simulink model "TwoD_Missile_Target"  (R2020b)
settings: Solver=ode4  StartTime=0.0  StopTime=simTime  FixedStep=h  MaxStep=h  RelTol=1e-3
values from neighbouring files (symbols this model uses):
  Beta = 0    [ProportionalNavigation.m]
  N_prime = 4    [ProportionalNavigation.m]
  nt = 3    [ProportionalNavigation.m]
  Rm1 = 0    [ProportionalNavigation.m]
  Rm2 = 10000    [ProportionalNavigation.m]
  Rt1 = 40000    [ProportionalNavigation.m]
  Rt2 = Rm2    (= 10000)    [ProportionalNavigation.m]
  Vm1_0 = Vm*cos(L+HE+Lambda)    [ProportionalNavigation.m]
  Vm2_0 = Vm*sin(L+HE+Lambda)    [ProportionalNavigation.m]
  Vt = 1000    [ProportionalNavigation.m]
  Vt1_0 = -Vt*cos(Beta)    [ProportionalNavigation.m]
  Vt2_0 = Vt*sin(Beta)    [ProportionalNavigation.m]
libraries: simulink x1
settings Model: Creator=dariusmensah  LastModifiedBy=dariusmensah
settings OptimizationCC: DefaultParameterBehavior=Inlined  EnhancedBackFolding=on  PassReuseOutputArgsAs=Individual arguments  ZeroExternalMemoryAtStartup=off  ZeroInternalMemoryAtStartup=off  OptimizeBlockOrder=speed  DifferentSizesBufferReuse=on  OptimizationCustomize=off  EfficientTunableParamExpr=on
settings DebuggingCC: ParameterTunabilityLossMsg=error
settings SFSimCC: MATLABDynamicMemAlloc=off
settings RTWCC: Description=Embedded Coder  SystemTargetFile=ert.tlc  TemplateMakefile=ert_default_tmf
settings CodeAppCC: ForceParamTrailComments=on  IgnoreCustomStorageClasses=off  OperatorAnnotations=on  SimulinkDataObjDesc=on  SFDataObjDesc=on  InsertBlockDesc=on
settings ERTTargetCC: TargetLangStandard=C99 (ISO)  GenerateSampleERTMain=on  SupportContinuousTime=on  InlinedParameterPlacement=NonHierarchical  ERTCustomFileTemplate=example_file_process.tlc

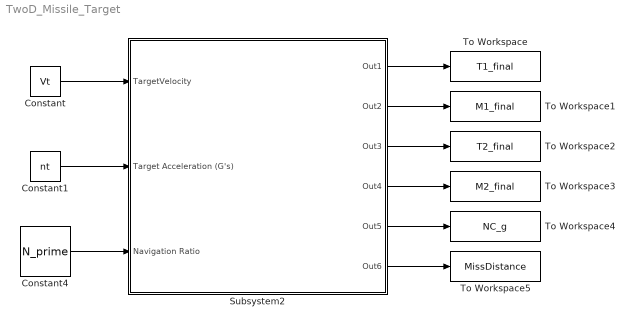
== system TwoD_Missile_Target ==
  Constant : Constant  Value=Vt
  Constant1 : Constant  Value=nt
  Constant4 : Constant  Value=N_prime
  Subsystem2 : Subsystem
  To Workspace : ToWorkspace  VariableName=T1_final  SaveFormat=Structure With Time  SampleTime=-1
  To Workspace1 : ToWorkspace  VariableName=M1_final  SaveFormat=Structure With Time  SampleTime=-1
  To Workspace2 : ToWorkspace  VariableName=T2_final  SaveFormat=Structure With Time  SampleTime=-1
  To Workspace3 : ToWorkspace  VariableName=M2_final  SaveFormat=Structure With Time  SampleTime=-1
  To Workspace4 : ToWorkspace  VariableName=NC_g  SaveFormat=Structure With Time  SampleTime=-1
  To Workspace5 : ToWorkspace  VariableName=MissDistance  SaveFormat=Structure With Time  SampleTime=-1
  wires:
  Subsystem2/2(Out2) -> To Workspace1/1
  Subsystem2/4(Out4) -> To Workspace3/1
  Constant/1 -> Subsystem2/1(TargetVelocity)
  Subsystem2/6(Out6) -> To Workspace5/1
  Constant4/1 -> Subsystem2/3(Navigation Ratio)
  Subsystem2/3(Out3) -> To Workspace2/1
  Subsystem2/5(Out5) -> To Workspace4/1
  Constant1/1 -> Subsystem2/2(Target Acceleration (G's))
  Subsystem2/1(Out1) -> To Workspace/1

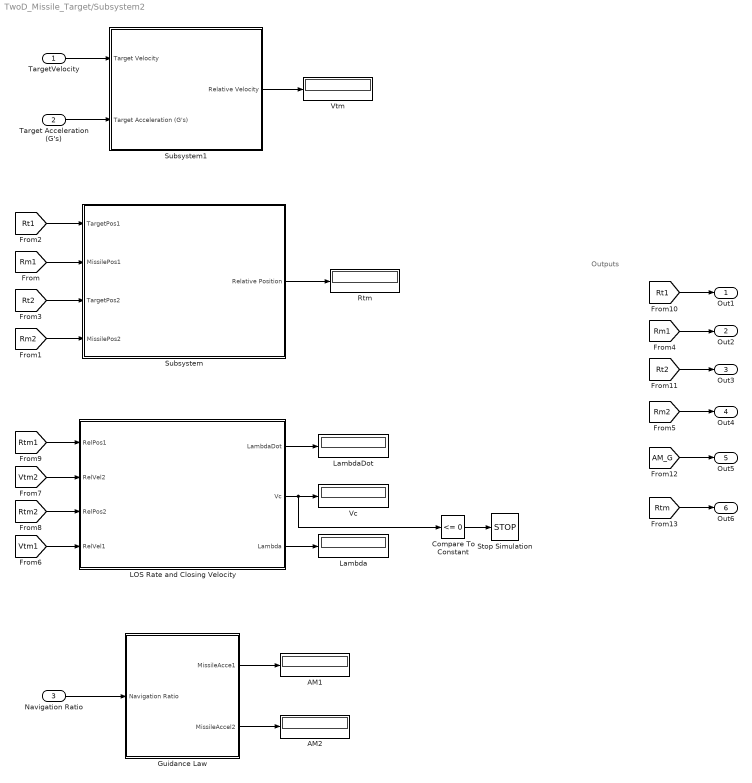
== system TwoD_Missile_Target/Subsystem2 ==
  note: Outputs
  TargetVelocity : Inport
  Target Acceleration (G's) : Inport  Port=2
  Navigation Ratio : Inport  Port=3
  AM1 : Display
  AM2 : Display
  Compare To Constant : simulink/Logic and Bit Operations/Compare To Constant  relop=<=  const=0  OutDataTypeStr=boolean
  Guidance Law : Subsystem
  LOS Rate and Closing Velocity : Subsystem
  Lambda : Display
  LambdaDot : Display
  Rtm : Display
  Stop Simulation : Stop
  Subsystem : Subsystem
  Subsystem1 : Subsystem
  Vc : Display
  Vtm : Display
  Out1 : Outport
  Out2 : Outport  Port=2
  Out3 : Outport  Port=3
  Out4 : Outport  Port=4
  Out5 : Outport  Port=5
  Out6 : Outport  Port=6
  wires:
  TargetVelocity/1 -> Subsystem1/1(Target Velocity)
  Navigation Ratio/1 -> Guidance Law/1(Navigation Ratio)
  [Vtm2] -> LOS Rate and Closing Velocity/2(RelVel2)
  [Rm2] -> Subsystem/4(MissilePos2)
  LOS Rate and Closing Velocity/1(LambdaDot) -> LambdaDot/1
  [Rt1] -> Subsystem/1(TargetPos1)
  [Rtm2] -> LOS Rate and Closing Velocity/3(RelPos2)
  [Rtm1] -> LOS Rate and Closing Velocity/1(RelPos1)
  Guidance Law/1(MissileAcce1) -> AM1/1
  [Vtm1] -> LOS Rate and Closing Velocity/4(RelVel1)
  Subsystem1/1(Relative Velocity) -> Vtm/1
  LOS Rate and Closing Velocity/2(Vc) -> Compare To Constant/1, Vc/1
  Guidance Law/2(MissileAccel2) -> AM2/1
  Subsystem/1(Relative Position) -> Rtm/1
  [Rt2] -> Subsystem/3(TargetPos2)
  LOS Rate and Closing Velocity/3(Lambda) -> Lambda/1
  [Rm1] -> Subsystem/2(MissilePos1)
  [Rt1] -> Out1/1
  [Rm2] -> Out4/1
  [Rm1] -> Out2/1
  [Rt2] -> Out3/1
  Compare To Constant/1 -> Stop Simulation/1
  [AM_G] -> Out5/1
  [Rtm] -> Out6/1
  Target Acceleration (G's)/1 -> Subsystem1/2(Target Acceleration (G's))

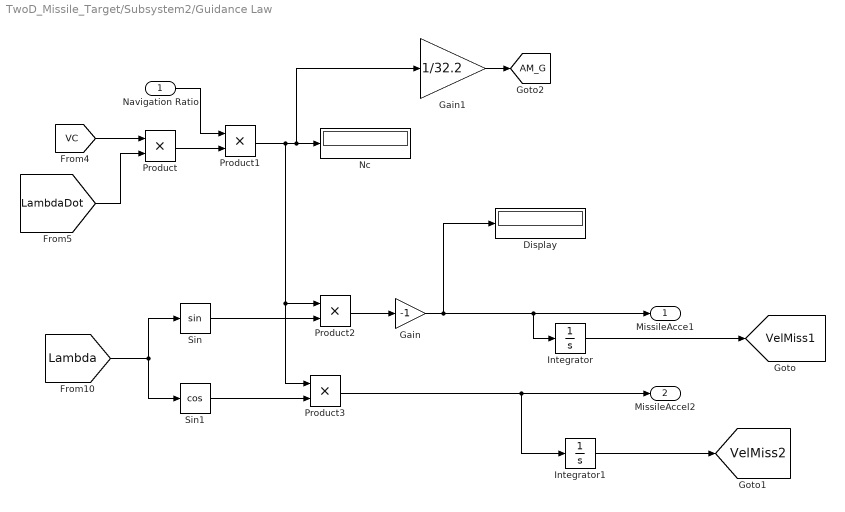
== system TwoD_Missile_Target/Subsystem2/Guidance Law ==
  Navigation Ratio : Inport
  Display : Display
  Gain : Gain  Gain=-1
  Gain1 : Gain  Gain=1/32.2
  Integrator : Integrator  InitialCondition=Vm1_0
  Integrator1 : Integrator  InitialCondition=Vm2_0
  Nc : Display
  Product{,1..3} (4 alike) : Product
  Sin : Trigonometry
  Sin1 : Trigonometry  Operator=cos
  MissileAcce1 : Outport
  MissileAccel2 : Outport  Port=2
  tag scope: AM_G=global, VelMiss1=global, VelMiss2=global
  wires:
  Sin/1 -> Product2/2
  Product3/1 -> Integrator1/1, MissileAccel2/1
  [LambdaDot] -> Product/2
  [Lambda] -> Sin/1, Sin1/1
  Product/1 -> Product1/2
  Product1/1 -> Product3/1, Product2/1, Gain1/1, Nc/1
  Sin1/1 -> Product3/2
  Gain/1 -> Display/1, Integrator/1, MissileAcce1/1
  [VC] -> Product/1
  Navigation Ratio/1 -> Product1/1
  Product2/1 -> Gain/1
  Integrator/1 -> [VelMiss1]
  Integrator1/1 -> [VelMiss2]
  Gain1/1 -> [AM_G]

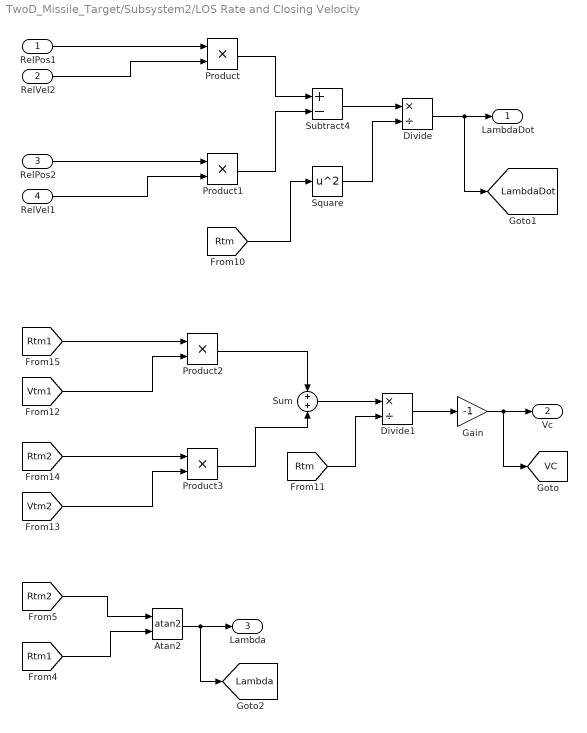
== system TwoD_Missile_Target/Subsystem2/LOS Rate and Closing Velocity ==
  RelPos1 : Inport
  RelVel2 : Inport  Port=2
  RelPos2 : Inport  Port=3
  RelVel1 : Inport  Port=4
  Atan2 : Trigonometry  Operator=atan2
  Divide : Product  Inputs=*/
  Divide1 : Product  Inputs=*/
  Gain : Gain  Gain=-1
  Product{,1..3} (4 alike) : Product
  Square : Math  Operator=square  SaturateOnIntegerOverflow=on
  Subtract4 : Sum  Inputs=+-
  Sum : Sum
  LambdaDot : Outport
  Vc : Outport  Port=2
  Lambda : Outport  Port=3
  tag scope: Lambda=global, LambdaDot=global, VC=global
  wires:
  RelVel2/1 -> Product/2
  RelPos1/1 -> Product/1
  [Vtm1] -> Product2/2
  Divide/1 -> [LambdaDot], LambdaDot/1
  Product2/1 -> Sum/1
  Square/1 -> Divide/2
  Product3/1 -> Sum/2
  Subtract4/1 -> Divide/1
  Product1/1 -> Subtract4/2
  Sum/1 -> Divide1/1
  [Rtm2] -> Product3/1
  [Vtm2] -> Product3/2
  [Rtm] -> Square/1
  [Rtm1] -> Product2/1
  RelVel1/1 -> Product1/2
  Gain/1 -> [VC], Vc/1
  RelPos2/1 -> Product1/1
  [Rtm] -> Divide1/2
  Product/1 -> Subtract4/1
  Divide1/1 -> Gain/1
  [Rtm2] -> Atan2/1
  [Rtm1] -> Atan2/2
  Atan2/1 -> [Lambda], Lambda/1

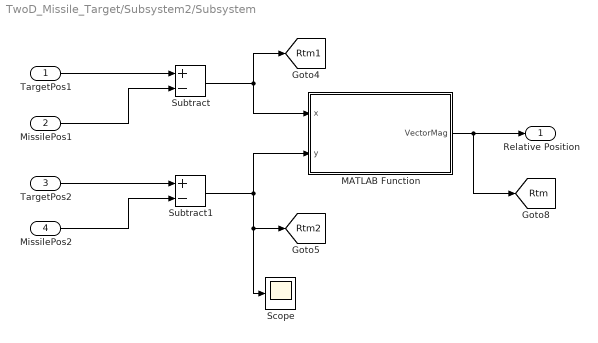
== system TwoD_Missile_Target/Subsystem2/Subsystem ==
  TargetPos1 : Inport
  MissilePos1 : Inport  Port=2
  TargetPos2 : Inport  Port=3
  MissilePos2 : Inport  Port=4
  MATLAB Function : MATLAB Function  TreatAsAtomicUnit=on
  Scope : Scope
  Subtract : Sum  Inputs=+-
  Subtract1 : Sum  Inputs=+-
  Relative Position : Outport
  tag scope: Rtm1=global, Rtm2=global, Rtm=global
  wires:
  MissilePos2/1 -> Subtract1/2
  MATLAB Function/1(VectorMag) -> Relative Position/1, [Rtm]
  Subtract1/1 -> Scope/1, [Rtm2], MATLAB Function/2(y)
  TargetPos1/1 -> Subtract/1
  TargetPos2/1 -> Subtract1/1
  Subtract/1 -> [Rtm1], MATLAB Function/1(x)
  MissilePos1/1 -> Subtract/2

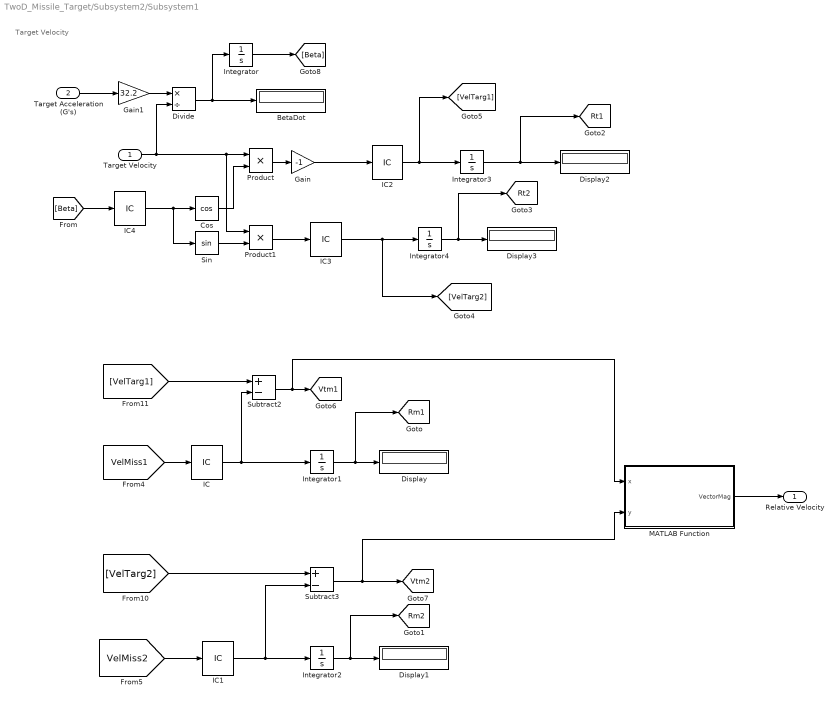
== system TwoD_Missile_Target/Subsystem2/Subsystem1 ==
  note: Target Velocity
  Target Velocity : Inport
  Target Acceleration (G's) : Inport  Port=2
  BetaDot : Display
  Cos : Trigonometry  Operator=cos
  Display{,1..3} (4 alike) : Display
  Divide : Product  Inputs=*/
  Gain : Gain  Gain=-1
  Gain1 : Gain  Gain=32.2
  IC : InitialCondition  Value=Vm1_0
  IC1 : InitialCondition  Value=Vm2_0
  IC2 : InitialCondition  Value=Vt1_0
  IC3 : InitialCondition  Value=Vt2_0
  IC4 : InitialCondition  Value=Beta
  Integrator : Integrator
  Integrator1 : Integrator  InitialCondition=Rm1
  Integrator2 : Integrator  InitialCondition=Rm2
  Integrator3 : Integrator  InitialCondition=Rt1
  Integrator4 : Integrator  InitialCondition=Rt2
  MATLAB Function : MATLAB Function  TreatAsAtomicUnit=on
  Product : Product
  Product1 : Product
  Sin : Trigonometry
  Subtract2 : Sum  Inputs=+-
  Subtract3 : Sum  Inputs=+-
  Relative Velocity : Outport
  tag scope: Rm1=global, Rm2=global, Rt1=global, Rt2=global, Vtm1=global, Vtm2=global
  wires:
  MATLAB Function/1(VectorMag) -> Relative Velocity/1
  [VelMiss1] -> IC/1
  Sin/1 -> Product1/2
  [VelTarg1] -> Subtract2/1
  Product/1 -> Gain/1
  Target Velocity/1 -> Divide/2, Product1/1, Product/1
  Subtract2/1 -> MATLAB Function/1(x), [Vtm1]
  [VelTarg2] -> Subtract3/1
  Cos/1 -> Product/2
  Product1/1 -> IC3/1
  Subtract3/1 -> MATLAB Function/2(y), [Vtm2]
  Integrator4/1 -> [Rt2], Display3/1
  IC/1 -> Integrator1/1, Subtract2/2
  [VelMiss2] -> IC1/1
  [Beta] -> IC4/1
  IC2/1 -> [VelTarg1], Integrator3/1
  Integrator2/1 -> [Rm2], Display1/1
  IC3/1 -> [VelTarg2], Integrator4/1
  Integrator1/1 -> [Rm1], Display/1
  Integrator3/1 -> Display2/1, [Rt1]
  IC1/1 -> Subtract3/2, Integrator2/1
  Gain/1 -> IC2/1
  Divide/1 -> BetaDot/1, Integrator/1
  IC4/1 -> Sin/1, Cos/1
  Integrator/1 -> [Beta]
  Target Acceleration (G's)/1 -> Gain1/1
  Gain1/1 -> Divide/1

== matlab function TwoD_Missile_Target/Subsystem2/Subsystem/MATLAB Function ==
  data: x input; VectorMag output; y input
function VectorMag = fcn(x,y)

a = x^2 + y^2;
VectorMag = sqrt(a);
end

== matlab function TwoD_Missile_Target/Subsystem2/Subsystem1/MATLAB Function ==
  data: x input; VectorMag output; y input
function VectorMag = fcn(x,y)

a = x^2 + y^2;
VectorMag = sqrt(a);
end
